simulink model "statespaceExSimulink1IntControl"  (R2023b)
settings: Solver=VariableStepAuto  StartTime=0.0  StopTime=10.0  RelTol=1e-3
undefined symbols (not defined in the file): A, B, C, K1, Ke
settings Model: Creator=klysm  LastModifiedBy=klysm

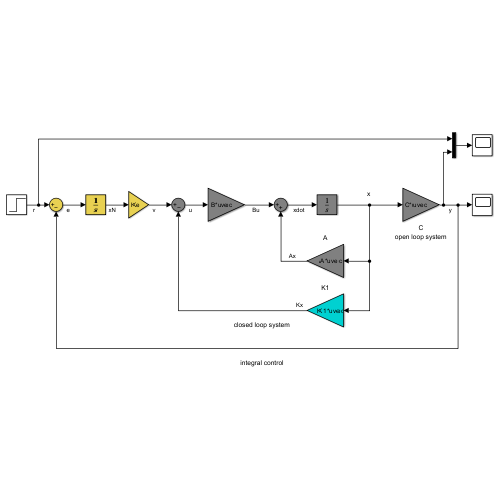
[thumbnail: Simulink's stored preview of the top-level diagram]
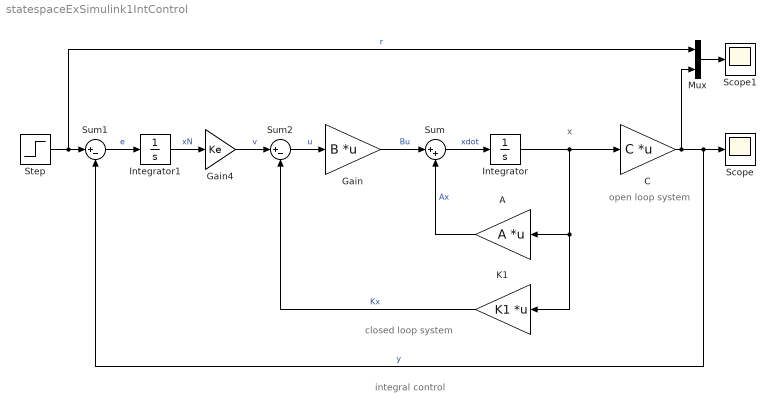
== system statespaceExSimulink1IntControl ==
  note: integral control
  note: x
  note: open loop system
  note: closed loop system
  A : Gain  Gain=A  Multiplication=Matrix(K*u) (u vector)
  C : Gain  Gain=C  Multiplication=Matrix(K*u) (u vector)
  Gain : Gain  Gain=B  Multiplication=Matrix(K*u) (u vector)
  Gain4 : Gain  Gain=Ke
  Integrator : Integrator
  Integrator1 : Integrator
  K1 : Gain  Gain=K1  Multiplication=Matrix(K*u) (u vector)
  Mux : Mux  Inputs=2
  Scope : Scope
  Scope1 : Scope
  Step : Step  SampleTime=0
  Sum : Sum  Inputs=|++
  Sum1 : Sum  Inputs=|+-
  Sum2 : Sum  Inputs=|+-
  wires:
  Sum/1 -> Integrator/1  "xdot"
  A/1 -> Sum/2  "Ax"
  Gain/1 -> Sum/1  "Bu"
  Integrator/1 -> C/1, K1/1, A/1
  C/1 -> Mux/2, Sum1/2, Scope/1  "y"
  Sum1/1 -> Integrator1/1  "e"
  K1/1 -> Sum2/2  "Kx"
  Step/1 -> Mux/1, Sum1/1  "r"
  Sum2/1 -> Gain/1  "u"
  Integrator1/1 -> Gain4/1  "xN"
  Gain4/1 -> Sum2/1  "v"
  Mux/1 -> Scope1/1
